simulink subsystem "RefPath"  (R2024b)
settings: Solver=VariableStepAuto  StartTime=0.0  StopTime=10.0  RelTol=1e-3
settings Model: Creator=Tong  LastModifiedBy=Tong

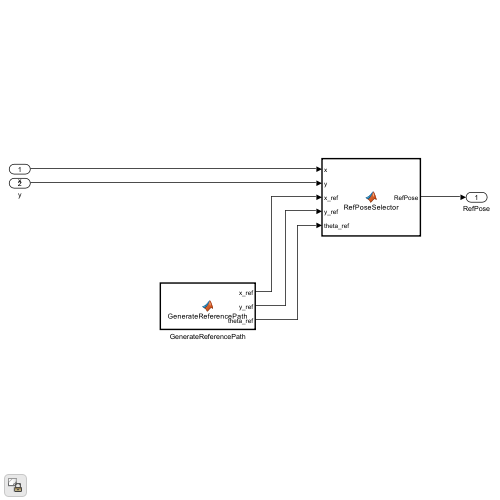
[thumbnail: Simulink's stored preview of the top-level diagram]
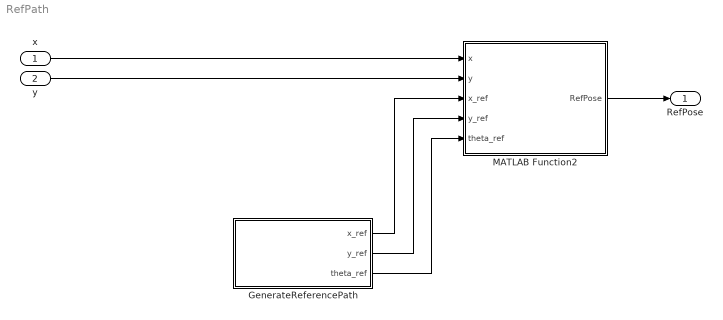
== system RefPath ==
  x : Inport
  y : Inport  Port=2
  GenerateReferencePath : MATLAB Function  TreatAsAtomicUnit=on
  MATLAB Function2 : MATLAB Function  TreatAsAtomicUnit=on
  RefPose : Outport
  wires:
  y/1 -> MATLAB Function2/2(y)
  MATLAB Function2/1(RefPose) -> RefPose/1
  GenerateReferencePath/1(x_ref) -> MATLAB Function2/3(x_ref)
  x/1 -> MATLAB Function2/1(x)
  GenerateReferencePath/2(y_ref) -> MATLAB Function2/4(y_ref)
  GenerateReferencePath/3(theta_ref) -> MATLAB Function2/5(theta_ref)

== matlab function RefPath/MATLAB Function2 ==
  settings: updateMethod=DISCRETE
  data: x input; RefPose output; y input; x_ref input; y_ref input; theta_ref input

% function RefPose = RefPoseSelector(x, y, x_ref, y_ref, theta_ref)
% % 根据当前车辆位置选择参考路径上的最近点
% %
% % 输入:
% %   x, y         - 当前车辆位置
% %   x_ref, y_ref - 参考路径坐标
% %   theta_ref    - 路径方向角（deg）
% %
% % 输出:
% %   RefPose      - [x_ref_i, y_ref_i, theta_ref_i]
% 
% dist = sqrt((x_ref - x).^2 + (y_ref - y).^2);
% [~, idx] = min(dist);
% 
% RefPose = [x_ref(idx), y_ref(idx), theta_ref(idx)];
% end


% function RefPose = RefPoseSelector(x, y, theta_deg, x_ref, y_ref, theta_ref)
% %#codegen
% % 工程版参考点选择：前轴选点 + 进度约束 + 预瞄
% %
% % 输入:
% %   x,y,theta_deg : 当前车辆后轴中心（或你CurrPose的点）与航向角(deg)
% %   x_ref,y_ref,theta_ref : 参考路径点与方向角
% % 输出:
% %   RefPose = [x_ref_i, y_ref_i, theta_ref_i]  (deg)
% 
% persistent idxLast
% if isempty(idxLast)
%     idxLast = 1;
% end
% 
% N = length(x_ref);
% 
% % ---- 参数（可调）----
% L = 2.8;            % 轴距（和Stanley块一致）
% win = 80;           % 搜索窗口（点数少就小一些；点数多就大一些）
% lookahead = 5;      % 预瞄点数（0~10都可试）
% % ---------------------
% 
% % 1) 用前轴中心选点（Stanley前进时的定义）
% xf = x + L*cosd(theta_deg);
% yf = y + L*sind(theta_deg);
% 
% % 2) 只在 idxLast 附近向前搜索，避免跳到其它路段
% i1 = idxLast;
% i2 = min(idxLast + win, N);
% 
% dx = x_ref(i1:i2) - xf;
% dy = y_ref(i1:i2) - yf;
% dist2 = dx.*dx + dy.*dy;
% 
% [~, k] = min(dist2);
% idx = i1 + k - 1;
% 
% % 3) 更新进度（不允许倒退）
% if idx < idxLast
%     idx = idxLast;
% end
% idxLast = idx;
% 
% % 4) 预瞄（让转向更平滑、更积极）
% idx2 = min(idx + lookahead, N);
% 
% RefPose = [x_ref(idx2), y_ref(idx2), theta_ref(idx2)];
% end


function RefPose = RefPoseSelector(x, y, x_ref, y_ref, theta_ref)
%#codegen
% 稳健版参考点选择：窗口搜索 + 允许回退 + 必要时回退全局最近点
% 适合点数少（例如29点）且避免选点跳变

persistent idxLast
if isempty(idxLast)
    idxLast = 1;
end

N = length(x_ref);

% ---- 参数（可调）----
win = 10;          % 点数少，窗口别太大（5~15）
distReset = 30;    % 若窗口内最近点距离>30m，就回退全局最近点
lookahead = 0;     % 先别预瞄（等跑稳再设 1~3）
% ---------------------

% 1) 在 idxLast 附近前后搜索（允许回退）
i1 = max(1, idxLast - win);
i2 = min(N, idxLast + win);

dx = x_ref(i1:i2) - x;
dy = y_ref(i1:i2) - y;
dist2 = dx.*dx + dy.*dy;

[minDist2, k] = min(dist2);
idx = i1 + k - 1;

% 2) 如果窗口内离得太远，说明窗口错位/初始化错，回退全局最近点
if sqrt(minDist2) > distReset
    dxg = x_ref - x;
    dyg = y_ref - y;
    [~, idx] = min(dxg.*dxg + dyg.*dyg);
end

idxLast = idx;

% 3) 预瞄（点少先用0，跑稳后再调）
idx2 = min(N, idx + lookahead);

RefPose = [x_ref(idx2), y_ref(idx2), theta_ref(idx2)];
end

== matlab function RefPath/GenerateReferencePath ==
  data: x_ref output; y_ref output; theta_ref output
% function [x_ref, y_ref, theta_ref] = GenerateReferencePath()
% %#codegen
% % 输出 ego 参考路径及路径方向角（deg）
% 
% egoWaypoints = [...
%    -227.25   -2.25    0.01;
%    -207.80   -2.20    0.00;
%    -190.30   -2.20    0.00;
%    -183.40   -0.80    0.00;
%    -182.20    8.90    0.00;
%    -184.10   22.20    0.00;
%    -187.90   40.60    0.00;
%    -196.70   63.00    0.00;
%    -200.00   84.50    0.00;
%    -200.20  100.80    0.00;
%    -200.20  105.30    0.00;
%    -198.41  106.64    0.00;
%    -192.12  106.48    0.00;
%    -178.48  106.17    0.00;
%    -166.71  106.48    0.00;
%    -151.74  106.13    0.00;
%    -135.50  106.00    0.00;
%    -123.00  106.20    0.00;
%    -117.90  106.39    0.00;
%    -116.30  106.20    0.00;
%    -115.32  103.81    0.00;
%    -114.90  99.90    0.00;
%    -114.00  88.30    0.00;
%    -114.50   76.70    0.00;
%    -114.50   62.80    0.00;
%    -114.20   52.60    0.00;
%    -114.70   42.00    0.00;
%    -114.70   33.70    0.00;
%    -114.50   10.10    0.00];
% 
% 
% 
% x_ref = egoWaypoints(:,1);
% y_ref = -egoWaypoints(:,2);
% 
% N = size(egoWaypoints,1);   % 29
% 
% theta_ref = zeros(N,1);
% theta_ref(1:N-1) = atan2d(diff(y_ref), diff(x_ref));
% theta_ref(N) = theta_ref(N-1);
% end

function [x_ref, y_ref, theta_ref] = GenerateReferencePath()
%#codegen
% 输出 ego 参考路径及路径方向角（deg）
egoWaypoints = [...
   -227.25   -2.25    0.01;
   -207.76   -2.49    0.00;
   -190.44   -1.97    0.00;
   -184.60    0.13    0.00;
   -182.20    8.90    0.00;
   -184.10   22.20    0.00;
   -188.36   39.62    0.00;
   -191.37   47.84    0.00;
   -196.70   63.00    0.00;
   -200.00   84.50    0.00;
   -200.20  100.80    0.00;
   -199.60  103.87    0.00;
   -198.53  105.27    0.00;
   -192.12  106.48    0.00;
   -178.48  106.17    0.00;
   -166.67  106.41    0.00;
   -151.74  106.13    0.00;
   -135.50  106.00    0.00;
   -123.56  106.29    0.00;
   -118.43  106.05    0.00;
   -116.48  105.26    0.00;
   -115.32  103.81    0.00;
   -114.68  100.14    0.00;
   -114.50   88.40    0.00;
   -114.50   76.70    0.00;
   -114.50   62.80    0.00;
   -114.47   52.61    0.00;
   -114.70   42.00    0.00;
   -114.70   33.70    0.00;
   -114.50   10.10    0.00;
   -113.63    4.27    0.00;
   -111.17    0.23    0.00;
   -108.40   -1.10    0.00;
   -103.00   -1.70    0.00;
   -96.45   -1.77    0.00;
   -88.60   -2.10    0.00;
   -77.90   -2.20    0.00;
   -67.60   -2.00    0.00;
   -58.70   -1.90    0.00;
   -50.30   -1.70    0.00;
   -43.70   -2.10    0.00;
   -35.60   -2.00    0.00;
   -29.20   -2.00    0.00;
   -20.70   -1.80    0.00;
   -13.80   -1.90    0.00;
   -9.15   -1.81    0.00;
   -3.55   -1.01    0.00;
   -0.60    1.10    0.00;
    2.80    1.90    0.00;
    6.50    1.90    0.00;
   11.51    1.88    0.00;
   16.52    2.11    0.00;
   22.09    2.09    0.00;
   28.75    2.05    0.00;
   34.78    2.32    0.00;
   38.90    2.34    0.00;
   44.15    2.47    0.00;
   48.39    1.94    0.00;
   51.50   -0.80    0.00;
   53.83   -1.67    0.00;
   60.20   -1.90    0.00;
   63.20   -1.80    0.00;
   70.60   -1.80    0.00];


x_ref = egoWaypoints(:,1);
y_ref = -egoWaypoints(:,2);

N = size(egoWaypoints,1);
theta_ref = zeros(N,1);
theta_ref(1:N-1) = atan2d(diff(y_ref), diff(x_ref));
theta_ref(N) = theta_ref(N-1);
end
